simulink model "mfcMU_quadra"  (R2015a)
settings: Solver=ode15s  StartTime=0.0  StopTime=4000  RelTol=1e-9  AbsTol=1e-12
InitFcn:
  | delta = 20;
  | kmu = 20000;
  | 
  | beta = 0;
  | %beta = -10;
  | gamma = 0;
  | gamma = 5;
  | 
  | dummy = 0;
  | 
  | Rinit = 30;
  | 
  | %mfcInit2 = [20.8395  498.2432    2.0000    0.0412];
  | mfcInit2 = [7.02293569736422 486.519388075139 1.89207954994663 0.0499959483398174];
  | 
  | %mfcInit1 = [20.8395  498.2432    2.0000    0.0412];
  | mfcInit1 = [7.02288203941727 486.519391407949 1.89207915898595 0.0499977006595934];
settings Model: Creator=ironi  LastModifiedBy=ironi
settings HardwareCC: ProdBitPerLong=64  ProdBitPerPointer=64  ProdWordSize=64  ProdHWDeviceType=Generic->64-bit Embedded Processor (LP64)

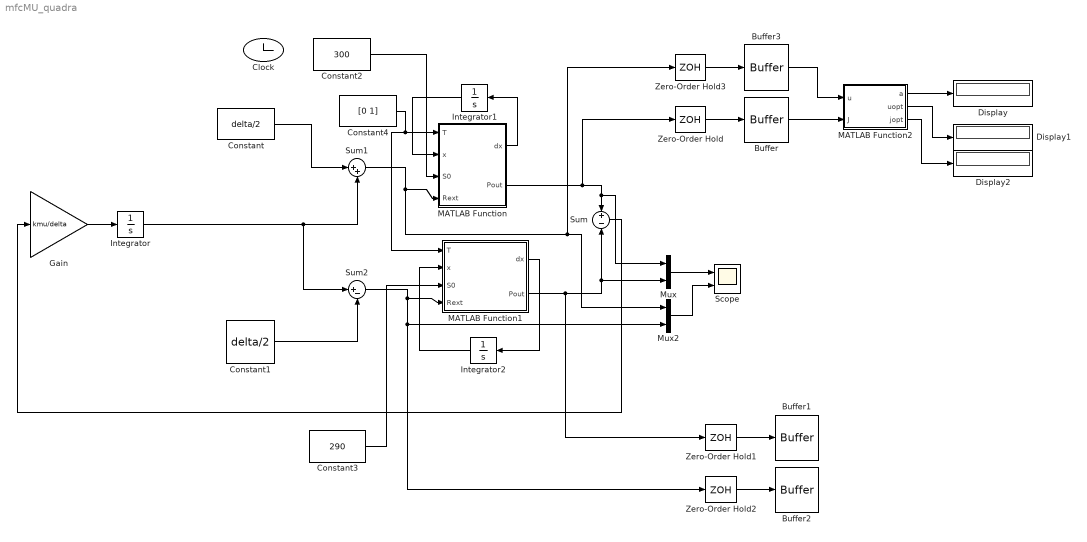
== system mfcMU_quadra ==
  Buffer{,1..3} (4 alike) : Buffer  N=3  TreatMby1Signals=One channel
  Clock : Clock
  Constant : Constant  Value=delta/2
  Constant1 : Constant  Value=delta/2
  Constant2 : Constant  Value=300
  Constant3 : Constant  Value=290
  Constant4 : Constant  Value=[0 1]
  Display : Display
  Display1 : Display
  Display2 : Display
  Gain : Gain  Gain=kmu/delta
  Integrator : Integrator  InitialCondition=Rinit
  Integrator1 : Integrator  InitialCondition=mfcInit2
  Integrator2 : Integrator  InitialCondition=mfcInit1
  MATLAB Function : MATLAB Function  TreatAsAtomicUnit=on
  MATLAB Function1 : MATLAB Function  TreatAsAtomicUnit=on
  MATLAB Function2 : MATLAB Function  TreatAsAtomicUnit=on
  Mux : Mux  Inputs=2
  Mux2 : Mux  Inputs=2
  Scope : Scope  NumInputPorts=2
      settings: YMin=0.00172~147  YMax=0.001734~168
  Sum : Sum  Inputs=+|-
  Sum1 : Sum  Inputs=|++
  Sum2 : Sum  Inputs=|+-
  Zero-Order Hold{,1..3} (4 alike) : ZeroOrderHold  SampleTime=.01
  wires:
  Sum/1 -> Gain/1
  Gain/1 -> Integrator/1
  Sum1/1 -> MATLAB Function/4(Rext), Zero-Order Hold3/1, Mux2/1
  Constant/1 -> Sum1/1
  Mux/1 -> Scope/1
  Constant1/1 -> Sum2/2
  Sum2/1 -> MATLAB Function1/4(Rext), Zero-Order Hold2/1, Mux2/2
  MATLAB Function/1(dx) -> Integrator1/1
  Mux2/1 -> Scope/2
  MATLAB Function/2(Pout) -> Zero-Order Hold/1, Mux/1, Sum/1
  Integrator1/1 -> MATLAB Function/2(x)
  MATLAB Function1/1(dx) -> Integrator2/1
  Constant4/1 -> MATLAB Function1/1(T), MATLAB Function/1(T)
  Constant2/1 -> MATLAB Function/3(S0)
  Constant3/1 -> MATLAB Function1/3(S0)
  Integrator/1 -> Sum2/1, Sum1/2
  Integrator2/1 -> MATLAB Function1/2(x)
  Zero-Order Hold/1 -> Buffer/1
  MATLAB Function1/2(Pout) -> Zero-Order Hold1/1, Mux/2, Sum/2
  Zero-Order Hold1/1 -> Buffer1/1
  Zero-Order Hold2/1 -> Buffer2/1
  Zero-Order Hold3/1 -> Buffer3/1
  Buffer3/1 -> MATLAB Function2/1(u)
  Buffer/1 -> MATLAB Function2/2(J)
  MATLAB Function2/1(a) -> Display/1
  MATLAB Function2/2(uopt) -> Display1/1
  MATLAB Function2/3(jopt) -> Display2/1

== matlab function mfcMU_quadra/MATLAB Function1 ==
  data: T input; dx output; x input; dummy parameter; S0 input; Rext input; Pout output
function [dx, Pout]= mfcModel(T, x, dummy, S0, Rext)
F = 96485;
R = 8.314472;
T = 298.15;
Y = 22.753;
Ych4 = .3;
qmax_a = 8.48;
qmax_m = 8.2;
umax_a = 1.9753;
umax_m = .1;
Ks_a = 20;
Ks_m = 80;
m = 2;
gamma = 663400;
Mtotal = .05;
Km = .2*Mtotal;
Kd_a = .02*umax_a;
Kd_m = .02*umax_m;
Xmax_a = 512.5;
Xmax_m = 537.5;
Kx = .04;
Rmin = 25;
Rmax = 2000 + Rmin;
Emin = .01;
Emax = 0.25 + 0.4144+ Emin;
Kr = .024;

i0ref=0.4*4;

e = 0.0001*Mtotal;

V = 0.05;
Fin = 0.1527;

D = Fin/V;

S   = x(1);
xa  = x(2);
xm  = x(3);
Mox = x(4);

%% Équations dynamiques
  
Mred = Mtotal - Mox;

Rint = Rmin + (Rmax - Rmin) * exp(-Kr*xa);                          % (22)
Eocv = Emin + (Emax - Emin) * exp(-1/(Kr*xa));                      % (23)

alpha_a = 1/2*(1 + tanh(Kx*(xa + xm - Xmax_a)));                    % (9)
alpha_m = 1/2*(1 + tanh(Kx*(xa + xm - Xmax_m)));                    % (9)

qa = qmax_a * S / (Ks_a + S) * Mox / (Km + Mox);                    % (15)
qm = qmax_m * S / (Ks_m + S);                                       % (16)

ua = umax_a * S / (Ks_a + S) * Mox / (Km + Mox);                    % (13)
um = umax_m * S / (Ks_m + S);                                       % (14)

n_conc = R*T/F/m * log(Mtotal/Mred);                                % (18)

Imfc = (Eocv - n_conc) / (Rext + Rint) * Mred / (e + Mred);         % (21)

Sp = -qa*xa - qm*xm + D*(S0 - S);                                   % (6)
Xap = ua*xa - Kd_a*xa - alpha_a*D*xa;                               % (7)
Xmp = um*xm - Kd_m*xm - alpha_m*D*xm;                               % (8)

Moxp = -Y*qa + gamma*Imfc / (m*F*V*xa) * 86400;                     % (12)

if xa < 1 && Xap < 0
  Xap = 0;
end

if xm < 0.99 && Xmp < 0
  Xmp = 0;
end

Pout = Rext*Imfc^2;

dx = [Sp; Xap; Xmp; Moxp];

== matlab function mfcMU_quadra/MATLAB Function ==
  data: T input; dx output; x input; dummy parameter; S0 input; Rext input; Pout output
function [dx, Pout]= mfcModel(T, x, dummy, S0, Rext)
F = 96485;
R = 8.314472;
T = 298.15;
Y = 22.753;
Ych4 = .3;
qmax_a = 8.48;
qmax_m = 8.2;
umax_a = 1.9753;
umax_m = .1;
Ks_a = 20;
Ks_m = 80;
m = 2;
gamma = 663400;
Mtotal = .05;
Km = .2*Mtotal;
Kd_a = .02*umax_a;
Kd_m = .02*umax_m;
Xmax_a = 512.5;
Xmax_m = 537.5;
Kx = .04;
Rmin = 25;
Rmax = 2000 + Rmin;
Emin = .01;
Emax = 0.25 + 0.4144+ Emin;
Kr = .024;

i0ref=0.4*4;

e = 0.0001*Mtotal;

V = 0.05;
Fin = 0.1527;

D = Fin/V;

S   = x(1);
xa  = x(2);
xm  = x(3);
Mox = x(4);

%% Équations dynamiques
  
Mred = Mtotal - Mox;

Rint = Rmin + (Rmax - Rmin) * exp(-Kr*xa);                          % (22)
Eocv = Emin + (Emax - Emin) * exp(-1/(Kr*xa));                      % (23)

alpha_a = 1/2*(1 + tanh(Kx*(xa + xm - Xmax_a)));                    % (9)
alpha_m = 1/2*(1 + tanh(Kx*(xa + xm - Xmax_m)));                    % (9)

qa = qmax_a * S / (Ks_a + S) * Mox / (Km + Mox);                    % (15)
qm = qmax_m * S / (Ks_m + S);                                       % (16)

ua = umax_a * S / (Ks_a + S) * Mox / (Km + Mox);                    % (13)
um = umax_m * S / (Ks_m + S);                                       % (14)

n_conc = R*T/F/m * log(Mtotal/Mred);                                % (18)

Imfc = (Eocv - n_conc) / (Rext + Rint) * Mred / (e + Mred);         % (21)

Sp = -qa*xa - qm*xm + D*(S0 - S);                                   % (6)
Xap = ua*xa - Kd_a*xa - alpha_a*D*xa;                               % (7)
Xmp = um*xm - Kd_m*xm - alpha_m*D*xm;                               % (8)

Moxp = -Y*qa + gamma*Imfc / (m*F*V*xa) * 86400;                     % (12)

if xa < 1 && Xap < 0
  Xap = 0;
end

if xm < 0.99 && Xmp < 0
  Xmp = 0;
end

Pout = Rext*Imfc^2;

dx = [Sp; Xap; Xmp; Moxp];

== matlab function mfcMU_quadra/MATLAB Function2 ==
  data: u input; a output; J input; uopt output; jopt output
function [a,uopt,jopt]= fcn(u,J)
%#codegen
% syms a uopt jopt
j1 = J(1);
j2 = J(2);
j3 = J(3);
u1 = u(1);
u2 = u(2);
u3 = u(3);

a = (j1*u2 - j2*u1 - j1*u3 + j3*u1 + j2*u3 - j3*u2)/((u1 - u2)*(u1*u2 - u1*u3 - u2*u3 + u3^2));

uopt = (j1*u2^2 - j2*u1^2 - j1*u3^2 + j3*u1^2 + j2*u3^2 - j3*u2^2)/(2*(j1*u2 - j2*u1 - j1*u3 + j3*u1 + j2*u3 - j3*u2));

jopt = -(j1^2*u2^4 - 4*j1^2*u2^3*u3 + 6*j1^2*u2^2*u3^2 - 4*j1^2*u2*u3^3 + j1^2*u3^4 - 2*j1*j2*u1^2*u2^2 + 4*j1*j2*u1^2*u2*u3 - 2*j1*j2*u1^2*u3^2 + 4*j1*j2*u1*u2^2*u3 - 8*j1*j2*u1*u2*u3^2 + 4*j1*j2*u1*u3^3 - 2*j1*j2*u2^2*u3^2 + 4*j1*j2*u2*u3^3 - 2*j1*j2*u3^4 - 2*j1*j3*u1^2*u2^2 + 4*j1*j3*u1^2*u2*u3 - 2*j1*j3*u1^2*u3^2 + 4*j1*j3*u1*u2^3 - 8*j1*j3*u1*u2^2*u3 + 4*j1*j3*u1*u2*u3^2 - 2*j1*j3*u2^4 + 4*j1*j3*u2^3*u3 - 2*j1*j3*u2^2*u3^2 + j2^2*u1^4 - 4*j2^2*u1^3*u3 + 6*j2^2*u1^2*u3^2 - 4*j2^2*u1*u3^3 + j2^2*u3^4 - 2*j2*j3*u1^4 + 4*j2*j3*u1^3*u2 + 4*j2*j3*u1^3*u3 - 2*j2*j3*u1^2*u2^2 - 8*j2*j3*u1^2*u2*u3 - 2*j2*j3*u1^2*u3^2 + 4*j2*j3*u1*u2^2*u3 + 4*j2*j3*u1*u2*u3^2 - 2*j2*j3*u2^2*u3^2 + j3^2*u1^4 - 4*j3^2*u1^3*u2 + 6*j3^2*u1^2*u2^2 - 4*j3^2*u1*u2^3 + j3^2*u2^4)/(4*(u1 - u2)*(u1*u2 - u1*u3 - u2*u3 + u3^2)*(j1*u2 - j2*u1 - j1*u3 + j3*u1 + j2*u3 - j3*u2));

% sys = solve( j(1) == a * (u(1) - uopt)^2 + jopt, ...
%              j(1) == a * (u(1) - uopt)^2 + jopt, ...
%              j(1) == a * (u(1) - uopt)^2 + jopt, ...
%              a, uopt, jopt);
% 
% a = double(sys.a);
% uopt = double(sys.uopt);
% jopt = double(sys.jopt);
